simulink model "x_square"  (R2018b)
settings: Solver=VariableStepAuto  StartTime=0.0  StopTime=10  RelTol=1e-3
settings Model: Creator=Administrator  LastModifiedBy=Administrator

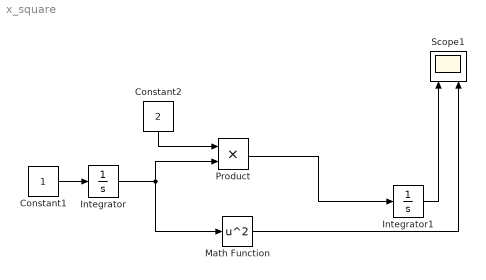
== system x_square ==
  Constant1 : Constant
  Constant2 : Constant  Value=2
  Integrator : Integrator  InitialCondition=eps
  Integrator1 : Integrator  InitialCondition=eps
  Math Function : Math  Operator=square  SaturateOnIntegerOverflow=on
  Product : Product
  Scope1 : Scope  NumInputPorts=2
  wires:
  Constant1/1 -> Integrator/1
  Product/1 -> Integrator1/1
  Integrator1/1 -> Scope1/1
  Math Function/1 -> Scope1/2
  Constant2/1 -> Product/1
  Integrator/1 -> Math Function/1, Product/2
